simulink model "Lab1Demo"  (Simulink 7.8)
settings: Solver=ode45  StartTime=0.0  StopTime=20  MaxStep=0.01  RelTol=1e-3
values from neighbouring files (symbols this model uses):
  b1 = .8    (= 0.8)    [Lab1DemoParam.m]
  b2 = .9    (= 0.9)    [Lab1DemoParam.m]
  b3 = .85    (= 0.85)    [Lab1DemoParam.m]
  k1 = 100    [Lab1DemoParam.m]
  k2 = 10    [Lab1DemoParam.m]
  k3 = 20    [Lab1DemoParam.m]
  m1 = .3    (= 0.3)    [Constants.m]    (also in Lab1DemoParam.m = 3)
  m2 = .05    (= 0.05)    [Constants.m]    (also in Lab1DemoParam.m = 2)
  X0 = [pi/2+.1 -.05 0 0]    [ABC.m]    (also in Constants.m = [pi/2 -pi 0 0]'; Lab1DemoParam.m = [.05 0 -.02 0])
settings Model: Creator=shahin  LastModifiedBy=salmas5
settings GRTTargetCC: CombineOutputUpdateFcns=on

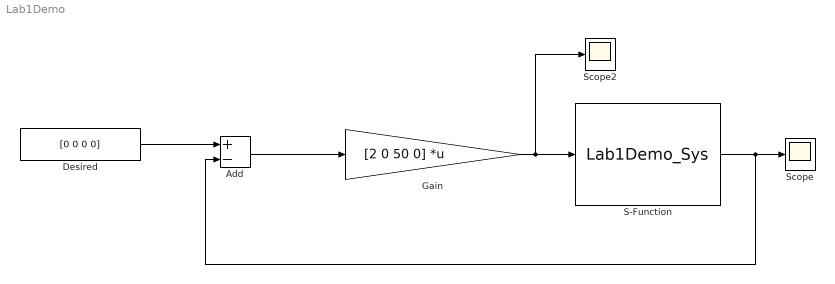
== system Lab1Demo ==
  Add : Sum  Inputs=+-
  "Desired " : Constant  Value=[0 0 0 0]
  Gain : Gain  Gain=[2 0 50 0]  Multiplication=Matrix(K*u)
  S-Function : S-Function  FunctionName=Lab1Demo_Sys  Parameters=X0,k1,k2,k3,b1,b2,b3,m1,m2  EnableBusSupport=off
  Scope : Scope
  Scope2 : Scope
      settings: SaveName=ScopeData2
  wires:
  Add/1 -> Gain/1
  Gain/1 -> S-Function/1, Scope2/1
  "Desired "/1 -> Add/1
  S-Function/1 -> Scope/1, Add/2
